simulink model "RockyBaseSystem"  (R2020b)
settings: Solver=VariableStepAuto  StartTime=0.0  StopTime=10.0  RelTol=1e-3
undefined symbols (not defined in the file): Ci, g, JiCp, Jp, K, Ki, Kp, L, tau
settings Model: Creator=nabih  LastModifiedBy=nabih

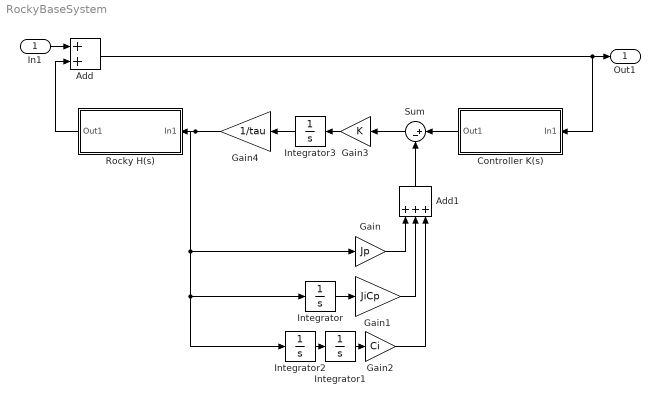
== system RockyBaseSystem ==
  In1 : Inport
  Add : Sum
  Add1 : Sum  Inputs=+++
  Controller K(s) : Subsystem
  Gain : Gain  Gain=Jp
  Gain1 : Gain  Gain=JiCp
  Gain2 : Gain  Gain=Ci
  Gain3 : Gain  Gain=K
  Gain4 : Gain  Gain=1/tau
  Integrator{,1..3} (4 alike) : Integrator
  Rocky H(s) : Subsystem
  Sum : Sum  Inputs=|+-
  Out1 : Outport
  wires:
  In1/1 -> Add/1
  Rocky H(s)/1(Out1) -> Add/2
  Add/1 -> Out1/1, Controller K(s)/1(In1)
  Controller K(s)/1(Out1) -> Sum/1
  Gain4/1 -> Gain/1, Integrator/1, Integrator2/1, Rocky H(s)/1(In1)
  Sum/1 -> Gain3/1
  Add1/1 -> Sum/2
  Integrator/1 -> Gain1/1
  Integrator1/1 -> Gain2/1
  Integrator2/1 -> Integrator1/1
  Gain2/1 -> Add1/3
  Gain1/1 -> Add1/2
  Gain/1 -> Add1/1
  Gain3/1 -> Integrator3/1
  Integrator3/1 -> Gain4/1

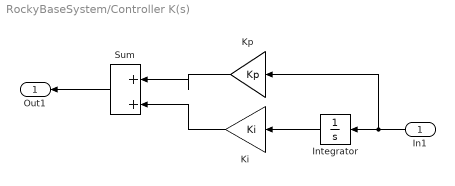
== system RockyBaseSystem/Controller K(s) ==
  In1 : Inport
  Integrator : Integrator
  Ki : Gain  Gain=Ki
  Kp : Gain  Gain=Kp
  Sum : Sum  Inputs=|++
  Out1 : Outport
  wires:
  Kp/1 -> Sum/1
  Ki/1 -> Sum/2
  Sum/1 -> Out1/1
  Integrator/1 -> Ki/1
  In1/1 -> Kp/1, Integrator/1

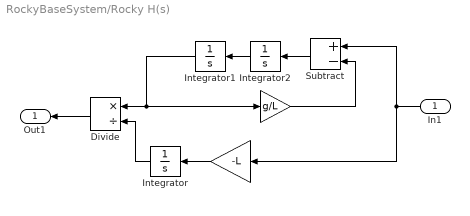
== system RockyBaseSystem/Rocky H(s) ==
  In1 : Inport
  " " : Gain  Gain=-L
  "  " : Gain  Gain=g/L
  Divide : Product  Inputs=*/
  Integrator : Integrator
  Integrator1 : Integrator
  Integrator2 : Integrator
  Subtract : Sum  Inputs=+-
  Out1 : Outport
  wires:
  In1/1 -> " "/1, Subtract/1
  Subtract/1 -> Integrator2/1
  "  "/1 -> Subtract/2
  Integrator1/1 -> Divide/1, "  "/1
  " "/1 -> Integrator/1
  Integrator2/1 -> Integrator1/1
  Integrator/1 -> Divide/2
  Divide/1 -> Out1/1
